simulink model "gtm_aeromodel"  (Simulink 7.2)
settings: Solver=ode45  StartTime=0.0  StopTime=10.0  RelTol=1e-3
undefined symbols (not defined in the file or in its folder): A_BLCG, A_BW, A_CW, A_FSCG, A_FSREF_in, A_SW, A_WLCG, A_WLREF, ALPHA0, bclowb, bclowbx_FMACH, bcmowb, bcmowbx_FHP, bcmowby_FMACH, cda, cdax_FLPDEF, cddr, cddrx_FMACH, cdo, cdox_FLPDEF, cdt1, cdt1x_mach, cdt2, cdt2x_mach, cdto, cdtox_mach, cdwb, cdwbx_FALPHA, cdwby_FMACH, clat, clatfr, clatfrx_FHP, clatfry_FMACH, clatx_mach, clawbfr, clawbfrx_FHP, clawbfry_FMACH, cldefr, cldefrx_FHP, cldefry_FMACH, cldtab, cldtabx_FMACH, clqwb, clqwbfr, clqwbfrx_FHP, clqwbfry_FMACH, clqwbx_mach, cltdd, cltddx_FHP, cltddy_FMACH, clwb, clwbtdd, clwbtddx_FHP, clwbtddy_FMACH, clwbx_FALPHA, clwby_FMACH, clwbzdd, clwbzddx_FHP, clwbzddy_FMACH, clzdd ... (+196)
libraries: model_lib x1
(part 6 of 10)

== system gtm_aeromodel/get aero forces and moments/AERODYNAMICS/Moment Coefficients/ROLL/CRR ==
  mach : Inport  OutDataType=sfix(16)  OutScaling=2^0
  alpha : Inport  Port=2  OutDataType=sfix(16)  OutScaling=2^0
  altitude : Inport  Port=3  OutDataType=sfix(16)  OutScaling=2^0
  flex : Inport  Port=4  OutDataType=sfix(16)  OutScaling=2^0
  rhat : Inport  Port=5  OutDataType=sfix(16)  OutScaling=2^0
  CRRFLEX : Subsystem  TreatAsAtomicUnit=on
  Fcn28 : Fcn  Expr=1/u
  Product2 : Product  Inputs=5  OutDataType=sfix(16)  OutScaling=2^0  SaturateOnIntegerOverflow=on  RndMeth=Zero  InputSameDT=on  OutDataTypeStr=Inherit: Same as first input
  Switch7 : Switch  Threshold=0.5  SaturateOnIntegerOverflow=on  InputSameDT=on
  constant : Constant  OutDataType=sfix(16)  OutScaling=2^0
  constant2 : Constant  Value=2  OutDataType=sfix(16)  OutScaling=2^0
  constant3 : Constant  Value=constants.r2d  OutDataType=sfix(16)  OutScaling=2^0
  crrtail : Product  OutDataType=sfix(16)  OutScaling=2^0  SaturateOnIntegerOverflow=on  RndMeth=Zero  InputSameDT=on  OutDataTypeStr=Inherit: Same as first input
  crrtot : Sum  Inputs=|++  OutDataType=sfix(16)  OutScaling=2^0  SaturateOnIntegerOverflow=on  InputSameDT=on  OutDataTypeStr=Inherit: Same as first input
  crrwb : Product  OutDataType=sfix(16)  OutScaling=2^0  SaturateOnIntegerOverflow=on  RndMeth=Zero  InputSameDT=on  OutDataTypeStr=Inherit: Same as first input
  crrwb_ : Subsystem  mask(2-D Table){y=crrwbx_FALPHA, z=crrwby_FMACH, tab=crrwb}
      mask prompts: y "Y vector:"; z "Z vector:"; tab "Table:"
      mask help: 2-D Table Look Up. Enter monotonic Y and Z vectors and a matrix of 2-D tables. See the help for more info.
      mask Help: The Y and Z vectors must be monotonic.  Y  indexes into the columns of the 2-D table & Z indexes into the rows of the 2-D tables.   The input values are y and z respectively (e.g., top port = y).
      mask Display: plot(-10,-10,110,110,[90,50,10],[90,40,30],[90,50,10],[50,26,20],[90,50,10],[22,13,10])
  dcyrt : Product  OutDataType=sfix(16)  OutScaling=2^0  SaturateOnIntegerOverflow=on  RndMeth=Zero  InputSameDT=on  OutDataTypeStr=Inherit: Same as first input
  rcnbvt : Subsystem  mask(2-D Table){y=cnbvtx_FMACH, z=cnbvty_FALPHA, tab=cnbvt}
      mask prompts: y "Y vector:"; z "Z vector:"; tab "Table:"
      mask help: 2-D Table Look Up. Enter monotonic Y and Z vectors and a matrix of 2-D tables. See the help for more info.
      mask Help: The Y and Z vectors must be monotonic.  Y  indexes into the columns of the 2-D table & Z indexes into the rows of the 2-D tables.   The input values are y and z respectively (e.g., top port = y).
      mask Display: plot(-10,-10,110,110,[90,50,10],[90,40,30],[90,50,10],[50,26,20],[90,50,10],[22,13,10])
  rcrbvt : Subsystem  mask(2-D Table){y=crbvtx_FMACH, z=crbvty_FALPHA, tab=crbvt}
      mask prompts: y "Y vector:"; z "Z vector:"; tab "Table:"
      mask help: 2-D Table Look Up. Enter monotonic Y and Z vectors and a matrix of 2-D tables. See the help for more info.
      mask Help: The Y and Z vectors must be monotonic.  Y  indexes into the columns of the 2-D table & Z indexes into the rows of the 2-D tables.   The input values are y and z respectively (e.g., top port = y).
      mask Display: plot(-10,-10,110,110,[90,50,10],[90,40,30],[90,50,10],[50,26,20],[90,50,10],[22,13,10])
  rcybvt : Subsystem  mask(2-D Table){y=cybvtx_FMACH, z=cybvty_FALPHA, tab=cybvt}
      mask prompts: y "Y vector:"; z "Z vector:"; tab "Table:"
      mask help: 2-D Table Look Up. Enter monotonic Y and Z vectors and a matrix of 2-D tables. See the help for more info.
      mask Help: The Y and Z vectors must be monotonic.  Y  indexes into the columns of the 2-D table & Z indexes into the rows of the 2-D tables.   The input values are y and z respectively (e.g., top port = y).
      mask Display: plot(-10,-10,110,110,[90,50,10],[90,40,30],[90,50,10],[50,26,20],[90,50,10],[22,13,10])
  dcrrhat : Outport  OutDataType=sfix(16)  OutScaling=2^0  InitialOutput=0
  wires:
  dcyrt/1 -> dcrrhat/1
  Switch7/1 -> crrwb/2, crrtail/2
  crrwb/1 -> crrtot/2
  crrwb_/1(Interp Value) -> crrwb/1
  rhat/1 -> dcyrt/2
  crrtot/1 -> dcyrt/1
  CRRFLEX/1(crrfr) -> Switch7/1
  constant/1 -> Switch7/3
  Product2/1 -> crrtail/1
  constant3/1 -> Product2/1
  rcrbvt/1(Interp Value) -> Product2/5
  Fcn28/1 -> Product2/3
  rcnbvt/1(Interp Value) -> Product2/2
  alpha/1 -> rcrbvt/2(Z), crrwb_/1(Y), rcybvt/2(Z), rcnbvt/2(Z)
  altitude/1 -> CRRFLEX/1(altitude)
  flex/1 -> CRRFLEX/Enable, Switch7/2
  mach/1 -> rcrbvt/1(Y), CRRFLEX/2(Mach), crrwb_/2(Z), rcnbvt/1(Y), rcybvt/1(Y)
  constant2/1 -> Product2/4
  rcybvt/1(Interp Value) -> Fcn28/1
  crrtail/1 -> crrtot/1

== system gtm_aeromodel/get aero forces and moments/AERODYNAMICS/Moment Coefficients/ROLL/CRRUD ==
  alpha : Inport  OutDataType=sfix(16)  OutScaling=2^0
  rud : Inport  Port=2  OutDataType=sfix(16)  OutScaling=2^0
  altitude : Inport  Port=3  OutDataType=sfix(16)  OutScaling=2^0
  flex : Inport  Port=4  OutDataType=sfix(16)  OutScaling=2^0
  mach : Inport  Port=5  OutDataType=sfix(16)  OutScaling=2^0
  CRFLEX : Subsystem  TreatAsAtomicUnit=on
  Product : Product  Inputs=3  OutDataType=sfix(16)  OutScaling=2^0  SaturateOnIntegerOverflow=on  RndMeth=Zero  InputSameDT=on  OutDataTypeStr=Inherit: Same as first input
  Switch7 : Switch  Threshold=0.5  SaturateOnIntegerOverflow=on  InputSameDT=on
  constant : Constant  OutDataType=sfix(16)  OutScaling=2^0
  crdr : Subsystem  mask(1-D Table){z=crdrx_FALPHA, tab=crdr}
      mask prompts: z "Z vector:"; tab "Table:"
      mask help: 1-D Table Look Up. Enter monotonic Z vector amd table. See the help for more info.
      mask Help: The Z vector must be monotonic.  Z indexes into the columns of the 1-D tables.   Table does not extrapolate beyound the break vectors
      mask Display: plot(@2)
  crrud : Outport  OutDataType=sfix(16)  OutScaling=2^0  InitialOutput=0
  wires:
  mach/1 -> CRFLEX/2(Mach)
  alpha/1 -> crdr/1(Z)
  crdr/1(Interp Value) -> Product/1
  rud/1 -> Product/2
  altitude/1 -> CRFLEX/1(altitude)
  Product/1 -> crrud/1
  Switch7/1 -> Product/3
  flex/1 -> CRFLEX/Enable, Switch7/2
  CRFLEX/1(crdrfr) -> Switch7/1
  constant/1 -> Switch7/3

== system gtm_aeromodel/get aero forces and moments/AERODYNAMICS/Moment Coefficients/ROLL/CRSPOIL ==
  dsb : Inport  OutDataType=sfix(16)  OutScaling=2^0
  dsl : Inport  Port=2  OutDataType=sfix(16)  OutScaling=2^0
  alpha : Inport  Port=3  OutDataType=sfix(16)  OutScaling=2^0
  mach : Inport  Port=4  OutDataType=sfix(16)  OutScaling=2^0
  flap : Inport  Port=5  OutDataType=sfix(16)  OutScaling=2^0
  altitude : Inport  Port=6  OutDataType=sfix(16)  OutScaling=2^0
  flex : Inport  Port=7  OutDataType=sfix(16)  OutScaling=2^0
  dsr : Inport  Port=8  OutDataType=sfix(16)  OutScaling=2^0
  MACH : Constant  Value=.178  OutDataType=sfix(16)  OutScaling=2^0
  Sum1 : Sum  Inputs=-+  OutDataType=sfix(16)  OutScaling=2^0  SaturateOnIntegerOverflow=on  InputSameDT=on  OutDataTypeStr=Inherit: Same as first input
  Sum10 : Sum  OutDataType=sfix(16)  OutScaling=2^0  SaturateOnIntegerOverflow=on  InputSameDT=on  OutDataTypeStr=Inherit: Same as first input
  Sum2 : Sum  Inputs=-+  OutDataType=sfix(16)  OutScaling=2^0  SaturateOnIntegerOverflow=on  InputSameDT=on  OutDataTypeStr=Inherit: Same as first input
  Sum{5..8} (4 alike) : Sum  Inputs=+-  OutDataType=sfix(16)  OutScaling=2^0  SaturateOnIntegerOverflow=on  InputSameDT=on  OutDataTypeStr=Inherit: Same as first input
  Sum9 : Sum  Inputs=-+  OutDataType=sfix(16)  OutScaling=2^0  SaturateOnIntegerOverflow=on  InputSameDT=on  OutDataTypeStr=Inherit: Same as first input
  Switch8 : Switch  Threshold=0.5  SaturateOnIntegerOverflow=on  InputSameDT=on
  Switch9 : Switch  Threshold=0.5  SaturateOnIntegerOverflow=on  InputSameDT=on
  cr_sp_fl : Subsystem  TreatAsAtomicUnit=on
  cr_sp_flex : Subsystem  TreatAsAtomicUnit=on
  dcrds : Product  OutDataType=sfix(16)  OutScaling=2^0  SaturateOnIntegerOverflow=on  RndMeth=Zero  InputSameDT=on  OutDataTypeStr=Inherit: Same as first input
  dcrwbdsbp : Subsystem  mask(1-2-3 Table){@1=dcrwbdslx_DSL, @2=dcrwbdsly_FALPHA, @3=dcrwbdslz_FMACH, @4=dcrwbdsl}
      mask prompts: @1 "X vector:"; @2 "Y vector:"; @3 "Z vector:"; @4 "Table:"
      mask help: 3-D Table Look Up. Enter monotonic X, Y and Z vectors and a matrix of 2-D tables. See the help for more info.
      mask init:
      | x=@1;y=@2;z=@3;tab=@4;
      mask Help: The X, Y and Z vectors must be monotonic.   The 3-D table is a horizontal concatenation of  2-D tables.  X  indexes into the columns of the 2-D tables & Y indexes into the rows of the 2-D tables.  Z indexes into the table levels (starting with the 1st 2-D table).   The input values are x, y and z respectively (e.g., top port = x).
      mask Display: plot([0 2 2 0 0],[0 0 2 2 0],[0 2 2.9 0.95 0],[2 2 2.7 2.7 2],[2 2.9 2.9 2 2],[0 0.85 2.7 2 0])
  dcrwbdsl : Subsystem  mask(1-2-3 Table){@1=dcrwbdslx_DSL, @2=dcrwbdsly_FALPHA, @3=dcrwbdslz_FMACH, @4=dcrwbdsl}
      mask prompts: @1 "X vector:"; @2 "Y vector:"; @3 "Z vector:"; @4 "Table:"
      mask help: 3-D Table Look Up. Enter monotonic X, Y and Z vectors and a matrix of 2-D tables. See the help for more info.
      mask init:
      | x=@1;y=@2;z=@3;tab=@4;
      mask Help: The X, Y and Z vectors must be monotonic.   The 3-D table is a horizontal concatenation of  2-D tables.  X  indexes into the columns of the 2-D tables & Y indexes into the rows of the 2-D tables.  Z indexes into the table levels (starting with the 1st 2-D table).   The input values are x, y and z respectively (e.g., top port = x).
      mask Display: plot([0 2 2 0 0],[0 0 2 2 0],[0 2 2.9 0.95 0],[2 2 2.7 2.7 2],[2 2.9 2.9 2 2],[0 0.85 2.7 2 0])
  dcrwbdsl1 : Subsystem  mask(1-2-3 Table){@1=dcrwbdslx_DSL, @2=dcrwbdsly_FALPHA, @3=dcrwbdslz_FMACH, @4=dcrwbdsl}
      mask prompts: @1 "X vector:"; @2 "Y vector:"; @3 "Z vector:"; @4 "Table:"
      mask help: 3-D Table Look Up. Enter monotonic X, Y and Z vectors and a matrix of 2-D tables. See the help for more info.
      mask init:
      | x=@1;y=@2;z=@3;tab=@4;
      mask Help: The X, Y and Z vectors must be monotonic.   The 3-D table is a horizontal concatenation of  2-D tables.  X  indexes into the columns of the 2-D tables & Y indexes into the rows of the 2-D tables.  Z indexes into the table levels (starting with the 1st 2-D table).   The input values are x, y and z respectively (e.g., top port = x).
      mask Display: plot([0 2 2 0 0],[0 0 2 2 0],[0 2 2.9 0.95 0],[2 2 2.7 2.7 2],[2 2.9 2.9 2 2],[0 0.85 2.7 2 0])
  dcrwbdsl2 : Subsystem  mask(1-2-3 Table){@1=dcrwbdslx_DSL, @2=dcrwbdsly_FALPHA, @3=dcrwbdslz_FMACH, @4=dcrwbdsl}
      mask prompts: @1 "X vector:"; @2 "Y vector:"; @3 "Z vector:"; @4 "Table:"
      mask help: 3-D Table Look Up. Enter monotonic X, Y and Z vectors and a matrix of 2-D tables. See the help for more info.
      mask init:
      | x=@1;y=@2;z=@3;tab=@4;
      mask Help: The X, Y and Z vectors must be monotonic.   The 3-D table is a horizontal concatenation of  2-D tables.  X  indexes into the columns of the 2-D tables & Y indexes into the rows of the 2-D tables.  Z indexes into the table levels (starting with the 1st 2-D table).   The input values are x, y and z respectively (e.g., top port = x).
      mask Display: plot([0 2 2 0 0],[0 0 2 2 0],[0 2 2.9 0.95 0],[2 2 2.7 2.7 2],[2 2.9 2.9 2 2],[0 0.85 2.7 2 0])
  dcrwbdsl3 : Subsystem  mask(1-2-3 Table){@1=dcrwbdslx_DSL, @2=dcrwbdsly_FALPHA, @3=dcrwbdslz_FMACH, @4=dcrwbdsl}
      mask prompts: @1 "X vector:"; @2 "Y vector:"; @3 "Z vector:"; @4 "Table:"
      mask help: 3-D Table Look Up. Enter monotonic X, Y and Z vectors and a matrix of 2-D tables. See the help for more info.
      mask init:
      | x=@1;y=@2;z=@3;tab=@4;
      mask Help: The X, Y and Z vectors must be monotonic.   The 3-D table is a horizontal concatenation of  2-D tables.  X  indexes into the columns of the 2-D tables & Y indexes into the rows of the 2-D tables.  Z indexes into the table levels (starting with the 1st 2-D table).   The input values are x, y and z respectively (e.g., top port = x).
      mask Display: plot([0 2 2 0 0],[0 0 2 2 0],[0 2 2.9 0.95 0],[2 2 2.7 2.7 2],[2 2.9 2.9 2 2],[0 0.85 2.7 2 0])
  dcrwbdsl4 : Subsystem  mask(1-2-3 Table){@1=dcrwbdslx_DSL, @2=dcrwbdsly_FALPHA, @3=dcrwbdslz_FMACH, @4=dcrwbdsl}
      mask prompts: @1 "X vector:"; @2 "Y vector:"; @3 "Z vector:"; @4 "Table:"
      mask help: 3-D Table Look Up. Enter monotonic X, Y and Z vectors and a matrix of 2-D tables. See the help for more info.
      mask init:
      | x=@1;y=@2;z=@3;tab=@4;
      mask Help: The X, Y and Z vectors must be monotonic.   The 3-D table is a horizontal concatenation of  2-D tables.  X  indexes into the columns of the 2-D tables & Y indexes into the rows of the 2-D tables.  Z indexes into the table levels (starting with the 1st 2-D table).   The input values are x, y and z respectively (e.g., top port = x).
      mask Display: plot([0 2 2 0 0],[0 0 2 2 0],[0 2 2.9 0.95 0],[2 2 2.7 2.7 2],[2 2.9 2.9 2 2],[0 0.85 2.7 2 0])
  one : Constant  Value=1.0  OutDataType=sfix(16)  OutScaling=2^0
  zero : Constant  Value=0.0  OutDataType=sfix(16)  OutScaling=2^0
  cr_spoil : Outport  OutDataType=sfix(16)  OutScaling=2^0  InitialOutput=0
  wires:
  dcrwbdsl/1(Interp Value) -> Sum1/2
  Sum10/1 -> cr_spoil/1
  alpha/1 -> dcrwbdsbp/2(Y), dcrwbdsl/2(Y), dcrwbdsl1/2(Y), dcrwbdsl3/2(Y), cr_sp_fl/2(alpha), dcrwbdsl4/2(Y), dcrwbdsl2/2(Y)
  dsl/1 -> dcrwbdsl/1(X), cr_sp_fl/3(dsl), dcrwbdsl3/1(X)
  dsb/1 -> dcrwbdsbp/1(X), cr_sp_fl/4(dsb), dcrwbdsl2/1(X)
  mach/1 -> dcrwbdsbp/3(Z), cr_sp_flex/2(mach), dcrwbdsl1/3(Z), dcrwbdsl/3(Z)
  altitude/1 -> cr_sp_flex/1(altitude)
  flap/1 -> cr_sp_fl/1(flap), cr_sp_fl/Enable, Switch8/2
  dcrwbdsl1/1(Interp Value) -> Sum5/1
  dcrwbdsbp/1(Interp Value) -> Sum1/1, Sum5/2
  Sum5/1 -> Sum6/2
  Sum6/1 -> dcrds/1
  dsr/1 -> dcrwbdsl1/1(X), dcrwbdsl4/1(X), cr_sp_fl/5(dsr)
  dcrwbdsl3/1(Interp Value) -> Sum2/2
  dcrwbdsl4/1(Interp Value) -> Sum7/1
  dcrwbdsl2/1(Interp Value) -> Sum2/1, Sum7/2
  Sum2/1 -> Sum8/1
  Sum7/1 -> Sum8/2
  MACH/1 -> dcrwbdsl2/3(Z), dcrwbdsl3/3(Z), dcrwbdsl4/3(Z)
  zero/1 -> Switch8/3
  cr_sp_fl/1(cr_sp_fl) -> Sum9/2
  Sum8/1 -> Sum9/1
  Sum9/1 -> Switch8/1
  Sum1/1 -> Sum6/1
  dcrds/1 -> Sum10/1
  Switch8/1 -> Sum10/2
  cr_sp_flex/1(cr_sp_flex) -> Switch9/1
  one/1 -> Switch9/3
  flex/1 -> cr_sp_flex/Enable, Switch9/2
  Switch9/1 -> dcrds/2

== system gtm_aeromodel/get aero forces and moments/AERODYNAMICS/Moment Coefficients/ROLL/TAIL ==
  mach : Inport  OutDataType=sfix(16)  OutScaling=2^0
  alpha : Inport  Port=2  OutDataType=sfix(16)  OutScaling=2^0
  Sum : Sum  OutDataType=sfix(16)  OutScaling=2^0  SaturateOnIntegerOverflow=on  InputSameDT=on  OutDataTypeStr=Inherit: Same as first input
  crbht : Subsystem  mask(2-D Table){y=crbhtx_FMACH, z=crbhty_FALPHA, tab=crbht}
      mask prompts: y "Y vector:"; z "Z vector:"; tab "Table:"
      mask help: 2-D Table Look Up. Enter monotonic Y and Z vectors and a matrix of 2-D tables. See the help for more info.
      mask Help: The Y and Z vectors must be monotonic.  Y  indexes into the columns of the 2-D table & Z indexes into the rows of the 2-D tables.   The input values are y and z respectively (e.g., top port = y).
      mask Display: plot(-10,-10,110,110,[90,50,10],[90,40,30],[90,50,10],[50,26,20],[90,50,10],[22,13,10])
  crbvt : Subsystem  mask(2-D Table){y=crbvtx_FMACH, z=crbvty_FALPHA, tab=crbvt}
      mask prompts: y "Y vector:"; z "Z vector:"; tab "Table:"
      mask help: 2-D Table Look Up. Enter monotonic Y and Z vectors and a matrix of 2-D tables. See the help for more info.
      mask Help: The Y and Z vectors must be monotonic.  Y  indexes into the columns of the 2-D table & Z indexes into the rows of the 2-D tables.   The input values are y and z respectively (e.g., top port = y).
      mask Display: plot(-10,-10,110,110,[90,50,10],[90,40,30],[90,50,10],[50,26,20],[90,50,10],[22,13,10])
  crt : Outport  OutDataType=sfix(16)  OutScaling=2^0  InitialOutput=0
  wires:
  crbvt/1(Interp Value) -> Sum/2
  Sum/1 -> crt/1
  crbht/1(Interp Value) -> Sum/1
  mach/1 -> crbht/1(Y), crbvt/1(Y)
  alpha/1 -> crbht/2(Z), crbvt/2(Z)

== system gtm_aeromodel/get aero forces and moments/AERODYNAMICS/Moment Coefficients/YAW/CNBWB ==
  alpha : Inport  OutDataType=sfix(16)  OutScaling=2^0
  mach : Inport  Port=2  OutDataType=sfix(16)  OutScaling=2^0
  flap : Inport  Port=3  OutDataType=sfix(16)  OutScaling=2^0
  flex : Inport  Port=4  OutDataType=sfix(16)  OutScaling=2^0
  altitude : Inport  Port=5  OutDataType=sfix(16)  OutScaling=2^0
  CNWBFLEX : Subsystem  TreatAsAtomicUnit=on
  Sum : Sum  OutDataType=sfix(16)  OutScaling=2^0  SaturateOnIntegerOverflow=on  InputSameDT=on  OutDataTypeStr=Inherit: Same as first input
  Switch5 : Switch  Threshold=0.1  SaturateOnIntegerOverflow=on  InputSameDT=on
  cn_flap_ : Subsystem  TreatAsAtomicUnit=on
  cnbwb_ : Subsystem  mask(2-D Table){y=cnbwbx_FMACH, z=cnbwby_FALPHA, tab=cnbwb}
      mask prompts: y "Y vector:"; z "Z vector:"; tab "Table:"
      mask help: 2-D Table Look Up. Enter monotonic Y and Z vectors and a matrix of 2-D tables. See the help for more info.
      mask Help: The Y and Z vectors must be monotonic.  Y  indexes into the columns of the 2-D table & Z indexes into the rows of the 2-D tables.   The input values are y and z respectively (e.g., top port = y).
      mask Display: plot(-10,-10,110,110,[90,50,10],[90,40,30],[90,50,10],[50,26,20],[90,50,10],[22,13,10])
  constant : Constant  Value=0.0  OutDataType=sfix(16)  OutScaling=2^0
  cnbwb : Outport  OutDataType=sfix(16)  OutScaling=2^0  InitialOutput=0
  cnbfr : Outport  Port=2  OutDataType=sfix(16)  OutScaling=2^0  InitialOutput=0
  wires:
  alpha/1 -> cn_flap_/2(alpha), cnbwb_/2(Z)
  Sum/1 -> cnbwb/1
  cnbwb_/1(Interp Value) -> Sum/2
  flap/1 -> cn_flap_/1(flap), cn_flap_/Enable, Switch5/2
  cn_flap_/1(cn_flap) -> Switch5/1
  altitude/1 -> CNWBFLEX/1(altitude)
  mach/1 -> cnbwb_/1(Y), CNWBFLEX/2(Mach)
  constant/1 -> Switch5/3
  Switch5/1 -> Sum/1
  flex/1 -> CNWBFLEX/Enable
  CNWBFLEX/1(cnbfr) -> cnbfr/1

== system gtm_aeromodel/get aero forces and moments/AERODYNAMICS/Moment Coefficients/YAW/CNGEAR ==
  flap : Inport  OutDataType=sfix(16)  OutScaling=2^0
  gear : Inport  Port=2  OutDataType=sfix(16)  OutScaling=2^0
  beta : Inport  Port=3  OutDataType=sfix(16)  OutScaling=2^0
  Product1 : Product  OutDataType=sfix(16)  OutScaling=2^0  SaturateOnIntegerOverflow=on  RndMeth=Zero  InputSameDT=on  OutDataTypeStr=Inherit: Same as first input
  Switch6 : Switch  Threshold=0.5  SaturateOnIntegerOverflow=on  InputSameDT=on
  constant1 : Constant  Value=0.0  OutDataType=sfix(16)  OutScaling=2^0
  dcnb : Subsystem  mask(1-D Table){z=dcnbx_FLPDEF, tab=dcnb}
      mask prompts: z "Z vector:"; tab "Table:"
      mask help: 1-D Table Look Up. Enter monotonic Z vector amd table. See the help for more info.
      mask Help: The Z vector must be monotonic.  Z indexes into the columns of the 1-D tables.   Table does not extrapolate beyound the break vectors
      mask Display: plot(@2)
  cng : Outport  OutDataType=sfix(16)  OutScaling=2^0  InitialOutput=0
  wires:
  Product1/1 -> Switch6/1
  beta/1 -> Product1/1
  Switch6/1 -> cng/1
  constant1/1 -> Switch6/3
  gear/1 -> Switch6/2
  flap/1 -> dcnb/1(Z)
  dcnb/1(Interp Value) -> Product1/2

== system gtm_aeromodel/get aero forces and moments/AERODYNAMICS/Moment Coefficients/YAW/CNP ==
  mach : Inport  OutDataType=sfix(16)  OutScaling=2^0
  alpha : Inport  Port=2  OutDataType=sfix(16)  OutScaling=2^0
  altitude : Inport  Port=3  OutDataType=sfix(16)  OutScaling=2^0
  flex : Inport  Port=4  OutDataType=sfix(16)  OutScaling=2^0
  phat : Inport  Port=5  OutDataType=sfix(16)  OutScaling=2^0
  CNPFLEX : Subsystem  TreatAsAtomicUnit=on
  Fcn28 : Fcn  Expr=1/u
  Product2 : Product  Inputs=5  OutDataType=sfix(16)  OutScaling=2^0  SaturateOnIntegerOverflow=on  RndMeth=Zero  InputSameDT=on  OutDataTypeStr=Inherit: Same as first input
  Switch7 : Switch  Threshold=0.5  SaturateOnIntegerOverflow=on  InputSameDT=on
  cnptail : Product  OutDataType=sfix(16)  OutScaling=2^0  SaturateOnIntegerOverflow=on  RndMeth=Zero  InputSameDT=on  OutDataTypeStr=Inherit: Same as first input
  cnptot : Sum  Inputs=|++  OutDataType=sfix(16)  OutScaling=2^0  SaturateOnIntegerOverflow=on  InputSameDT=on  OutDataTypeStr=Inherit: Same as first input
  cnpwb : Product  OutDataType=sfix(16)  OutScaling=2^0  SaturateOnIntegerOverflow=on  RndMeth=Zero  InputSameDT=on  OutDataTypeStr=Inherit: Same as first input
  constant : Constant  OutDataType=sfix(16)  OutScaling=2^0
  constant2 : Constant  Value=2  OutDataType=sfix(16)  OutScaling=2^0
  constant3 : Constant  Value=constants.r2d  OutDataType=sfix(16)  OutScaling=2^0
  dcyrt : Product  OutDataType=sfix(16)  OutScaling=2^0  SaturateOnIntegerOverflow=on  RndMeth=Zero  InputSameDT=on  OutDataTypeStr=Inherit: Same as first input
  rcnbvt : Subsystem  mask(2-D Table){y=cnbvtx_FMACH, z=cnbvty_FALPHA, tab=cnbvt}
      mask prompts: y "Y vector:"; z "Z vector:"; tab "Table:"
      mask help: 2-D Table Look Up. Enter monotonic Y and Z vectors and a matrix of 2-D tables. See the help for more info.
      mask Help: The Y and Z vectors must be monotonic.  Y  indexes into the columns of the 2-D table & Z indexes into the rows of the 2-D tables.   The input values are y and z respectively (e.g., top port = y).
      mask Display: plot(-10,-10,110,110,[90,50,10],[90,40,30],[90,50,10],[50,26,20],[90,50,10],[22,13,10])
  rcnpwb : Subsystem  mask(2-D Table){y=cnpwbx_FMACH, z=cnpwby_FALPHA, tab=cnpwb}
      mask prompts: y "Y vector:"; z "Z vector:"; tab "Table:"
      mask help: 2-D Table Look Up. Enter monotonic Y and Z vectors and a matrix of 2-D tables. See the help for more info.
      mask Help: The Y and Z vectors must be monotonic.  Y  indexes into the columns of the 2-D table & Z indexes into the rows of the 2-D tables.   The input values are y and z respectively (e.g., top port = y).
      mask Display: plot(-10,-10,110,110,[90,50,10],[90,40,30],[90,50,10],[50,26,20],[90,50,10],[22,13,10])
  rcrbvt : Subsystem  mask(2-D Table){y=crbvtx_FMACH, z=crbvty_FALPHA, tab=crbvt}
      mask prompts: y "Y vector:"; z "Z vector:"; tab "Table:"
      mask help: 2-D Table Look Up. Enter monotonic Y and Z vectors and a matrix of 2-D tables. See the help for more info.
      mask Help: The Y and Z vectors must be monotonic.  Y  indexes into the columns of the 2-D table & Z indexes into the rows of the 2-D tables.   The input values are y and z respectively (e.g., top port = y).
      mask Display: plot(-10,-10,110,110,[90,50,10],[90,40,30],[90,50,10],[50,26,20],[90,50,10],[22,13,10])
  rcybvt : Subsystem  mask(2-D Table){y=cybvtx_FMACH, z=cybvty_FALPHA, tab=cybvt}
      mask prompts: y "Y vector:"; z "Z vector:"; tab "Table:"
      mask help: 2-D Table Look Up. Enter monotonic Y and Z vectors and a matrix of 2-D tables. See the help for more info.
      mask Help: The Y and Z vectors must be monotonic.  Y  indexes into the columns of the 2-D table & Z indexes into the rows of the 2-D tables.   The input values are y and z respectively (e.g., top port = y).
      mask Display: plot(-10,-10,110,110,[90,50,10],[90,40,30],[90,50,10],[50,26,20],[90,50,10],[22,13,10])
  dcnphat : Outport  Orientation=left  OutDataType=sfix(16)  OutScaling=2^0  InitialOutput=0
  wires:
  constant3/1 -> Product2/1
  rcnbvt/1(Interp Value) -> Product2/5
  rcybvt/1(Interp Value) -> Fcn28/1
  rcrbvt/1(Interp Value) -> Product2/2
  Switch7/1 -> cnpwb/2, cnptail/2
  cnpwb/1 -> cnptot/2
  rcnpwb/1(Interp Value) -> cnpwb/1
  constant/1 -> Switch7/3
  CNPFLEX/1(cnpfr) -> Switch7/1
  Product2/1 -> cnptail/1
  cnptot/1 -> dcyrt/1
  phat/1 -> dcyrt/2
  cnptail/1 -> cnptot/1
  constant2/1 -> Product2/4
  mach/1 -> rcnbvt/1(Y), rcnpwb/1(Y), CNPFLEX/2(Mach), rcybvt/1(Y), rcrbvt/1(Y)
  flex/1 -> Switch7/2, CNPFLEX/Enable
  altitude/1 -> CNPFLEX/1(altitude)
  alpha/1 -> rcnbvt/2(Z), rcybvt/2(Z), rcrbvt/2(Z), rcnpwb/2(Z)
  Fcn28/1 -> Product2/3
  dcyrt/1 -> dcnphat/1

== system gtm_aeromodel/get aero forces and moments/AERODYNAMICS/Moment Coefficients/YAW/CNR ==
  mach : Inport  OutDataType=sfix(16)  OutScaling=2^0
  alpha : Inport  Port=2  OutDataType=sfix(16)  OutScaling=2^0
  altitude : Inport  Port=3  OutDataType=sfix(16)  OutScaling=2^0
  flex : Inport  Port=4  OutDataType=sfix(16)  OutScaling=2^0
  rhat : Inport  Port=5  OutDataType=sfix(16)  OutScaling=2^0
  CNRFLEX : Subsystem  TreatAsAtomicUnit=on
  Fcn28 : Fcn  Expr=1/u
  Product2 : Product  Inputs=4  OutDataType=sfix(16)  OutScaling=2^0  SaturateOnIntegerOverflow=on  RndMeth=Zero  InputSameDT=on  OutDataTypeStr=Inherit: Same as first input
  Product3 : Product  OutDataType=sfix(16)  OutScaling=2^0  SaturateOnIntegerOverflow=on  RndMeth=Zero  InputSameDT=on  OutDataTypeStr=Inherit: Same as first input
  Switch7 : Switch  Threshold=0.5  SaturateOnIntegerOverflow=on  InputSameDT=on
  cnrtail : Product  OutDataType=sfix(16)  OutScaling=2^0  SaturateOnIntegerOverflow=on  RndMeth=Zero  InputSameDT=on  OutDataTypeStr=Inherit: Same as first input
  cnrtot : Sum  Inputs=|++  OutDataType=sfix(16)  OutScaling=2^0  SaturateOnIntegerOverflow=on  InputSameDT=on  OutDataTypeStr=Inherit: Same as first input
  cnrwb : Product  OutDataType=sfix(16)  OutScaling=2^0  SaturateOnIntegerOverflow=on  RndMeth=Zero  InputSameDT=on  OutDataTypeStr=Inherit: Same as first input
  constant : Constant  OutDataType=sfix(16)  OutScaling=2^0
  constant2 : Constant  Value=2  OutDataType=sfix(16)  OutScaling=2^0
  constant3 : Constant  Value=constants.r2d  OutDataType=sfix(16)  OutScaling=2^0
  dcyrt : Product  OutDataType=sfix(16)  OutScaling=2^0  SaturateOnIntegerOverflow=on  RndMeth=Zero  InputSameDT=on  OutDataTypeStr=Inherit: Same as first input
  rcnbvt : Subsystem  mask(2-D Table){y=cnbvtx_FMACH, z=cnbvty_FALPHA, tab=cnbvt}
      mask prompts: y "Y vector:"; z "Z vector:"; tab "Table:"
      mask help: 2-D Table Look Up. Enter monotonic Y and Z vectors and a matrix of 2-D tables. See the help for more info.
      mask Help: The Y and Z vectors must be monotonic.  Y  indexes into the columns of the 2-D table & Z indexes into the rows of the 2-D tables.   The input values are y and z respectively (e.g., top port = y).
      mask Display: plot(-10,-10,110,110,[90,50,10],[90,40,30],[90,50,10],[50,26,20],[90,50,10],[22,13,10])
  rcnrwb : Subsystem  mask(2-D Table){y=cnrwbx_FALPHA, z=cnrwby_FMACH, tab=cnrwb}
      mask prompts: y "Y vector:"; z "Z vector:"; tab "Table:"
      mask help: 2-D Table Look Up. Enter monotonic Y and Z vectors and a matrix of 2-D tables. See the help for more info.
      mask Help: The Y and Z vectors must be monotonic.  Y  indexes into the columns of the 2-D table & Z indexes into the rows of the 2-D tables.   The input values are y and z respectively (e.g., top port = y).
      mask Display: plot(-10,-10,110,110,[90,50,10],[90,40,30],[90,50,10],[50,26,20],[90,50,10],[22,13,10])
  rcybvt : Subsystem  mask(2-D Table){y=cybvtx_FMACH, z=cybvty_FALPHA, tab=cybvt}
      mask prompts: y "Y vector:"; z "Z vector:"; tab "Table:"
      mask help: 2-D Table Look Up. Enter monotonic Y and Z vectors and a matrix of 2-D tables. See the help for more info.
      mask Help: The Y and Z vectors must be monotonic.  Y  indexes into the columns of the 2-D table & Z indexes into the rows of the 2-D tables.   The input values are y and z respectively (e.g., top port = y).
      mask Display: plot(-10,-10,110,110,[90,50,10],[90,40,30],[90,50,10],[50,26,20],[90,50,10],[22,13,10])
  dcnrhat : Outport  OutDataType=sfix(16)  OutScaling=2^0  InitialOutput=0
  wires:
  constant3/1 -> Product2/1
  Switch7/1 -> cnrwb/2, cnrtail/2
  constant/1 -> Switch7/3
  CNRFLEX/1(cnrfr) -> Switch7/1
  Product3/1 -> Product2/2
  rcnbvt/1(Interp Value) -> Product3/2, Product3/1
  cnrwb/1 -> cnrtot/2
  rcnrwb/1(Interp Value) -> cnrwb/1
  Product2/1 -> cnrtail/1
  dcyrt/1 -> dcnrhat/1
  cnrtot/1 -> dcyrt/1
  rhat/1 -> dcyrt/2
  cnrtail/1 -> cnrtot/1
  rcybvt/1(Interp Value) -> Fcn28/1
  constant2/1 -> Product2/4
  mach/1 -> rcnrwb/2(Z), CNRFLEX/2(Mach), rcybvt/1(Y), rcnbvt/1(Y)
  flex/1 -> Switch7/2, CNRFLEX/Enable
  altitude/1 -> CNRFLEX/1(altitude)
  alpha/1 -> rcnbvt/2(Z), rcybvt/2(Z), rcnrwb/1(Y)
  Fcn28/1 -> Product2/3

== system gtm_aeromodel/get aero forces and moments/AERODYNAMICS/Moment Coefficients/YAW/CNRUD ==
  rud : Inport  OutDataType=sfix(16)  OutScaling=2^0
  altitude : Inport  Port=2  OutDataType=sfix(16)  OutScaling=2^0
  flex : Inport  Port=3  OutDataType=sfix(16)  OutScaling=2^0
  mach : Inport  Port=4  OutDataType=sfix(16)  OutScaling=2^0
  CNFLEX : Subsystem  TreatAsAtomicUnit=on
  Product : Product  Inputs=3  OutDataType=sfix(16)  OutScaling=2^0  SaturateOnIntegerOverflow=on  RndMeth=Zero  InputSameDT=on  OutDataTypeStr=Inherit: Same as first input
  Switch7 : Switch  Threshold=0.5  SaturateOnIntegerOverflow=on  InputSameDT=on
  cndr : Subsystem  mask(1-D Table){z=cndrx_FMACH, tab=cndr}
      mask prompts: z "Z vector:"; tab "Table:"
      mask help: 1-D Table Look Up. Enter monotonic Z vector amd table. See the help for more info.
      mask Help: The Z vector must be monotonic.  Z indexes into the columns of the 1-D tables.   Table does not extrapolate beyound the break vectors
      mask Display: plot(@2)
  constant : Constant  OutDataType=sfix(16)  OutScaling=2^0
  cnrud : Outport  OutDataType=sfix(16)  OutScaling=2^0  InitialOutput=0
  wires:
  mach/1 -> cndr/1(Z), CNFLEX/2(Mach)
  constant/1 -> Switch7/3
  CNFLEX/1(cndrfr) -> Switch7/1
  flex/1 -> Switch7/2, CNFLEX/Enable
  Switch7/1 -> Product/3
  Product/1 -> cnrud/1
  altitude/1 -> CNFLEX/1(altitude)
  rud/1 -> Product/2
  cndr/1(Interp Value) -> Product/1

== system gtm_aeromodel/get aero forces and moments/AERODYNAMICS/Moment Coefficients/YAW/CNSPOIL ==
  dsb : Inport  OutDataType=sfix(16)  OutScaling=2^0
  dsl : Inport  Port=2  OutDataType=sfix(16)  OutScaling=2^0
  alpha : Inport  Port=3  OutDataType=sfix(16)  OutScaling=2^0
  mach : Inport  Port=4  OutDataType=sfix(16)  OutScaling=2^0
  flap : Inport  Port=5  OutDataType=sfix(16)  OutScaling=2^0
  dsr : Inport  Port=6  OutDataType=sfix(16)  OutScaling=2^0
  MACH : Constant  Value=.178  OutDataType=sfix(16)  OutScaling=2^0
  Sum1 : Sum  Inputs=-+  OutDataType=sfix(16)  OutScaling=2^0  SaturateOnIntegerOverflow=on  InputSameDT=on  OutDataTypeStr=Inherit: Same as first input
  Sum10 : Sum  OutDataType=sfix(16)  OutScaling=2^0  SaturateOnIntegerOverflow=on  InputSameDT=on  OutDataTypeStr=Inherit: Same as first input
  Sum2 : Sum  Inputs=-+  OutDataType=sfix(16)  OutScaling=2^0  SaturateOnIntegerOverflow=on  InputSameDT=on  OutDataTypeStr=Inherit: Same as first input
  Sum{5..8} (4 alike) : Sum  Inputs=+-  OutDataType=sfix(16)  OutScaling=2^0  SaturateOnIntegerOverflow=on  InputSameDT=on  OutDataTypeStr=Inherit: Same as first input
  Sum9 : Sum  Inputs=-+  OutDataType=sfix(16)  OutScaling=2^0  SaturateOnIntegerOverflow=on  InputSameDT=on  OutDataTypeStr=Inherit: Same as first input
  Switch8 : Switch  Threshold=0.5  SaturateOnIntegerOverflow=on  InputSameDT=on
  cn_sp_fl : Subsystem  TreatAsAtomicUnit=on
  dcnwbdsl : Subsystem  mask(1-2-3 Table){@1=dcnwbdslx_DSL, @2=dcnwbdsly_FALPHA, @3=dcnwbdslz_FMACH, @4=dcnwbdsl}
      mask prompts: @1 "X vector:"; @2 "Y vector:"; @3 "Z vector:"; @4 "Table:"
      mask help: 3-D Table Look Up. Enter monotonic X, Y and Z vectors and a matrix of 2-D tables. See the help for more info.
      mask init:
      | x=@1;y=@2;z=@3;tab=@4;
      mask Help: The X, Y and Z vectors must be monotonic.   The 3-D table is a horizontal concatenation of  2-D tables.  X  indexes into the columns of the 2-D tables & Y indexes into the rows of the 2-D tables.  Z indexes into the table levels (starting with the 1st 2-D table).   The input values are x, y and z respectively (e.g., top port = x).
      mask Display: plot([0 2 2 0 0],[0 0 2 2 0],[0 2 2.9 0.95 0],[2 2 2.7 2.7 2],[2 2.9 2.9 2 2],[0 0.85 2.7 2 0])
  dcnwbdsl1 : Subsystem  mask(1-2-3 Table){@1=dcnwbdslx_DSL, @2=dcnwbdsly_FALPHA, @3=dcnwbdslz_FMACH, @4=dcnwbdsl}
      mask prompts: @1 "X vector:"; @2 "Y vector:"; @3 "Z vector:"; @4 "Table:"
      mask help: 3-D Table Look Up. Enter monotonic X, Y and Z vectors and a matrix of 2-D tables. See the help for more info.
      mask init:
      | x=@1;y=@2;z=@3;tab=@4;
      mask Help: The X, Y and Z vectors must be monotonic.   The 3-D table is a horizontal concatenation of  2-D tables.  X  indexes into the columns of the 2-D tables & Y indexes into the rows of the 2-D tables.  Z indexes into the table levels (starting with the 1st 2-D table).   The input values are x, y and z respectively (e.g., top port = x).
      mask Display: plot([0 2 2 0 0],[0 0 2 2 0],[0 2 2.9 0.95 0],[2 2 2.7 2.7 2],[2 2.9 2.9 2 2],[0 0.85 2.7 2 0])
  dcnwbdsl2 : Subsystem  mask(1-2-3 Table){@1=dcnwbdslx_DSL, @2=dcnwbdsly_FALPHA, @3=dcnwbdslz_FMACH, @4=dcnwbdsl}
      mask prompts: @1 "X vector:"; @2 "Y vector:"; @3 "Z vector:"; @4 "Table:"
      mask help: 3-D Table Look Up. Enter monotonic X, Y and Z vectors and a matrix of 2-D tables. See the help for more info.
      mask init:
      | x=@1;y=@2;z=@3;tab=@4;
      mask Help: The X, Y and Z vectors must be monotonic.   The 3-D table is a horizontal concatenation of  2-D tables.  X  indexes into the columns of the 2-D tables & Y indexes into the rows of the 2-D tables.  Z indexes into the table levels (starting with the 1st 2-D table).   The input values are x, y and z respectively (e.g., top port = x).
      mask Display: plot([0 2 2 0 0],[0 0 2 2 0],[0 2 2.9 0.95 0],[2 2 2.7 2.7 2],[2 2.9 2.9 2 2],[0 0.85 2.7 2 0])
  dcnwbdsl3 : Subsystem  mask(1-2-3 Table){@1=dcnwbdslx_DSL, @2=dcnwbdsly_FALPHA, @3=dcnwbdslz_FMACH, @4=dcnwbdsl}
      mask prompts: @1 "X vector:"; @2 "Y vector:"; @3 "Z vector:"; @4 "Table:"
      mask help: 3-D Table Look Up. Enter monotonic X, Y and Z vectors and a matrix of 2-D tables. See the help for more info.
      mask init:
      | x=@1;y=@2;z=@3;tab=@4;
      mask Help: The X, Y and Z vectors must be monotonic.   The 3-D table is a horizontal concatenation of  2-D tables.  X  indexes into the columns of the 2-D tables & Y indexes into the rows of the 2-D tables.  Z indexes into the table levels (starting with the 1st 2-D table).   The input values are x, y and z respectively (e.g., top port = x).
      mask Display: plot([0 2 2 0 0],[0 0 2 2 0],[0 2 2.9 0.95 0],[2 2 2.7 2.7 2],[2 2.9 2.9 2 2],[0 0.85 2.7 2 0])
  dcnwbdsl4 : Subsystem  mask(1-2-3 Table){@1=dcnwbdslx_DSL, @2=dcnwbdsly_FALPHA, @3=dcnwbdslz_FMACH, @4=dcnwbdsl}
      mask prompts: @1 "X vector:"; @2 "Y vector:"; @3 "Z vector:"; @4 "Table:"
      mask help: 3-D Table Look Up. Enter monotonic X, Y and Z vectors and a matrix of 2-D tables. See the help for more info.
      mask init:
      | x=@1;y=@2;z=@3;tab=@4;
      mask Help: The X, Y and Z vectors must be monotonic.   The 3-D table is a horizontal concatenation of  2-D tables.  X  indexes into the columns of the 2-D tables & Y indexes into the rows of the 2-D tables.  Z indexes into the table levels (starting with the 1st 2-D table).   The input values are x, y and z respectively (e.g., top port = x).
      mask Display: plot([0 2 2 0 0],[0 0 2 2 0],[0 2 2.9 0.95 0],[2 2 2.7 2.7 2],[2 2.9 2.9 2 2],[0 0.85 2.7 2 0])
  dcnwbdsl5 : Subsystem  mask(1-2-3 Table){@1=dcnwbdslx_DSL, @2=dcnwbdsly_FALPHA, @3=dcnwbdslz_FMACH, @4=dcnwbdsl}
      mask prompts: @1 "X vector:"; @2 "Y vector:"; @3 "Z vector:"; @4 "Table:"
      mask help: 3-D Table Look Up. Enter monotonic X, Y and Z vectors and a matrix of 2-D tables. See the help for more info.
      mask init:
      | x=@1;y=@2;z=@3;tab=@4;
      mask Help: The X, Y and Z vectors must be monotonic.   The 3-D table is a horizontal concatenation of  2-D tables.  X  indexes into the columns of the 2-D tables & Y indexes into the rows of the 2-D tables.  Z indexes into the table levels (starting with the 1st 2-D table).   The input values are x, y and z respectively (e.g., top port = x).
      mask Display: plot([0 2 2 0 0],[0 0 2 2 0],[0 2 2.9 0.95 0],[2 2 2.7 2.7 2],[2 2.9 2.9 2 2],[0 0.85 2.7 2 0])
  zero : Constant  Value=0.0  OutDataType=sfix(16)  OutScaling=2^0
  cn_spoil : Outport  Orientation=left  OutDataType=sfix(16)  OutScaling=2^0  InitialOutput=0
  wires:
  Switch8/1 -> Sum10/2
  Sum1/1 -> Sum6/1
  Sum9/1 -> Switch8/1
  Sum8/1 -> Sum9/1
  cn_sp_fl/1(cn_sp_fl) -> Sum9/2
  zero/1 -> Switch8/3
  MACH/1 -> dcnwbdsl5/3(Z), dcnwbdsl4/3(Z), dcnwbdsl3/3(Z)
  Sum7/1 -> Sum8/2
  Sum2/1 -> Sum8/1
  dcnwbdsl3/1(Interp Value) -> Sum7/2, Sum2/1
  dcnwbdsl5/1(Interp Value) -> Sum7/1
  dcnwbdsl4/1(Interp Value) -> Sum2/2
  dsr/1 -> cn_sp_fl/5(dsr), dcnwbdsl5/1(X), dcnwbdsl2/1(X)
  Sum5/1 -> Sum6/2
  dcnwbdsl/1(Interp Value) -> Sum5/2, Sum1/1
  dcnwbdsl2/1(Interp Value) -> Sum5/1
  flap/1 -> Switch8/2, cn_sp_fl/Enable, cn_sp_fl/1(flap)
  mach/1 -> dcnwbdsl1/3(Z), dcnwbdsl/3(Z), dcnwbdsl2/3(Z)
  dsb/1 -> dcnwbdsl3/1(X), cn_sp_fl/4(dsb), dcnwbdsl/1(X)
  dsl/1 -> dcnwbdsl4/1(X), cn_sp_fl/3(dsl), dcnwbdsl1/1(X)
  alpha/1 -> dcnwbdsl3/2(Y), dcnwbdsl5/2(Y), cn_sp_fl/2(alpha), dcnwbdsl4/2(Y), dcnwbdsl2/2(Y), dcnwbdsl1/2(Y), dcnwbdsl/2(Y)
  Sum10/1 -> cn_spoil/1
  dcnwbdsl1/1(Interp Value) -> Sum1/2
  Sum6/1 -> Sum10/1

== system gtm_aeromodel/get aero forces and moments/AERODYNAMICS/Moment Coefficients/YAW/CNT ==
  mach : Inport  OutDataType=sfix(16)  OutScaling=2^0
  alpha : Inport  Port=2  OutDataType=sfix(16)  OutScaling=2^0
  Sum : Sum  OutDataType=sfix(16)  OutScaling=2^0  SaturateOnIntegerOverflow=on  InputSameDT=on  OutDataTypeStr=Inherit: Same as first input
  cnbht : Subsystem  mask(2-D Table){y=cnbhtx_FMACH, z=cnbhty_FALPHA, tab=cnbht}
      mask prompts: y "Y vector:"; z "Z vector:"; tab "Table:"
      mask help: 2-D Table Look Up. Enter monotonic Y and Z vectors and a matrix of 2-D tables. See the help for more info.
      mask Help: The Y and Z vectors must be monotonic.  Y  indexes into the columns of the 2-D table & Z indexes into the rows of the 2-D tables.   The input values are y and z respectively (e.g., top port = y).
      mask Display: plot(-10,-10,110,110,[90,50,10],[90,40,30],[90,50,10],[50,26,20],[90,50,10],[22,13,10])
  cnbvt : Subsystem  mask(2-D Table){y=cnbvtx_FMACH, z=cnbvty_FALPHA, tab=cnbvt}
      mask prompts: y "Y vector:"; z "Z vector:"; tab "Table:"
      mask help: 2-D Table Look Up. Enter monotonic Y and Z vectors and a matrix of 2-D tables. See the help for more info.
      mask Help: The Y and Z vectors must be monotonic.  Y  indexes into the columns of the 2-D table & Z indexes into the rows of the 2-D tables.   The input values are y and z respectively (e.g., top port = y).
      mask Display: plot(-10,-10,110,110,[90,50,10],[90,40,30],[90,50,10],[50,26,20],[90,50,10],[22,13,10])
  cnt : Outport  OutDataType=sfix(16)  OutScaling=2^0  InitialOutput=0
  wires:
  alpha/1 -> cnbvt/2(Z), cnbht/2(Z)
  mach/1 -> cnbvt/1(Y), cnbht/1(Y)
  cnbht/1(Interp Value) -> Sum/1
  Sum/1 -> cnt/1
  cnbvt/1(Interp Value) -> Sum/2

== system gtm_aeromodel/get aero forces and moments/AERODYNAMICS/Aero Incidence Angles/DOWNWASH/deps_hob_/depshob_ ==
  X : Inport  OutDataType=sfix(16)  OutScaling=2^0
  Y : Inport  Port=2  OutDataType=sfix(16)  OutScaling=2^0
  Z : Inport  Port=3  OutDataType=sfix(16)  OutScaling=2^0
  Mux : Mux  Inputs=3
  S-Function : S-Function  FunctionName=table3v5  Parameters=x,y,z,tab  EnableBusSupport=off
  Interp Value : Outport  OutDataType=sfix(16)  OutScaling=2^0
  wires:
  Z/1 -> Mux/3
  Y/1 -> Mux/2
  X/1 -> Mux/1
  Mux/1 -> S-Function/1
  S-Function/1 -> Interp Value/1

== system gtm_aeromodel/get aero forces and moments/AERODYNAMICS/Aero Incidence Angles/DOWNWASH/depsct/gbct ==
  Z : Inport  OutDataType=sfix(16)  OutScaling=2^0
  S-Function : S-Function  FunctionName=table1v5  Parameters=z,tab  EnableBusSupport=off
  Interp Value : Outport  OutDataType=sfix(16)  OutScaling=2^0
  wires:
  Z/1 -> S-Function/1
  S-Function/1 -> Interp Value/1

== system gtm_aeromodel/get aero forces and moments/AERODYNAMICS/Aero Incidence Angles/DOWNWASH/eps_flap/dclwbdffr ==
  qdyn : Inport  OutDataType=sfix(16)  OutScaling=2^0
  flap : Inport  Port=2  OutDataType=sfix(16)  OutScaling=2^0
  Enable : EnablePort
  dclwbdffr_ : Subsystem  mask(2-D Table){y=dclwbdffrx_FQ, z=dclwbdffry_FLPDEF, tab=dclwbdffr}
      mask prompts: y "Y vector:"; z "Z vector:"; tab "Table:"
      mask help: 2-D Table Look Up. Enter monotonic Y and Z vectors and a matrix of 2-D tables. See the help for more info.
      mask Help: The Y and Z vectors must be monotonic.  Y  indexes into the columns of the 2-D table & Z indexes into the rows of the 2-D tables.   The input values are y and z respectively (e.g., top port = y).
      mask Display: plot(-10,-10,110,110,[90,50,10],[90,40,30],[90,50,10],[50,26,20],[90,50,10],[22,13,10])
  dclwbdffr : Outport  OutDataType=sfix(16)  OutScaling=2^0  InitialOutput=0
  wires:
  dclwbdffr_/1(Interp Value) -> dclwbdffr/1
  qdyn/1 -> dclwbdffr_/1(Y)
  flap/1 -> dclwbdffr_/2(Z)

== system gtm_aeromodel/get aero forces and moments/AERODYNAMICS/Aero Incidence Angles/DOWNWASH/eps_flap/epsa ==
  Z : Inport  OutDataType=sfix(16)  OutScaling=2^0
  S-Function : S-Function  FunctionName=table1v5  Parameters=z,tab  EnableBusSupport=off
  Interp Value : Outport  OutDataType=sfix(16)  OutScaling=2^0
  wires:
  S-Function/1 -> Interp Value/1
  Z/1 -> S-Function/1

== system gtm_aeromodel/get aero forces and moments/AERODYNAMICS/Aero Incidence Angles/DOWNWASH/eps_flap/epsdsbdf ==
  X : Inport  OutDataType=sfix(16)  OutScaling=2^0
  Y : Inport  Port=2  OutDataType=sfix(16)  OutScaling=2^0
  Z : Inport  Port=3  OutDataType=sfix(16)  OutScaling=2^0
  Mux : Mux  Inputs=3
  S-Function : S-Function  FunctionName=table3v5  Parameters=x,y,z,tab  EnableBusSupport=off
  Interp Value : Outport  OutDataType=sfix(16)  OutScaling=2^0
  wires:
  Z/1 -> Mux/3
  Y/1 -> Mux/2
  X/1 -> Mux/1
  Mux/1 -> S-Function/1
  S-Function/1 -> Interp Value/1

== system gtm_aeromodel/get aero forces and moments/AERODYNAMICS/Aero Incidence Angles/DOWNWASH/eps_flap/epsodsb ==
  Y : Inport  OutDataType=sfix(16)  OutScaling=2^0
  Z : Inport  Port=2  OutDataType=sfix(16)  OutScaling=2^0
  Mux : Mux  Inputs=2
  S-Function : S-Function  FunctionName=table2v5  Parameters=y,z,tab  EnableBusSupport=off
  Interp Value : Outport  OutDataType=sfix(16)  OutScaling=2^0
  wires:
  Z/1 -> Mux/2
  Y/1 -> Mux/1
  S-Function/1 -> Interp Value/1
  Mux/1 -> S-Function/1

== system gtm_aeromodel/get aero forces and moments/AERODYNAMICS/Aero Incidence Angles/DOWNWASH/eps_speedbrake_/epsodsb ==
  Y : Inport  OutDataType=sfix(16)  OutScaling=2^0
  Z : Inport  Port=2  OutDataType=sfix(16)  OutScaling=2^0
  Mux : Mux  Inputs=2
  S-Function : S-Function  FunctionName=table2v5  Parameters=y,z,tab  EnableBusSupport=off
  Interp Value : Outport  OutDataType=sfix(16)  OutScaling=2^0
  wires:
  Z/1 -> Mux/2
  Y/1 -> Mux/1
  S-Function/1 -> Interp Value/1
  Mux/1 -> S-Function/1

== system gtm_aeromodel/get aero forces and moments/AERODYNAMICS/Aero Incidence Angles/DOWNWASH/eps_speedbrake_/epsodsb_0 ==
  Y : Inport  OutDataType=sfix(16)  OutScaling=2^0
  Z : Inport  Port=2  OutDataType=sfix(16)  OutScaling=2^0
  Mux : Mux  Inputs=2
  S-Function : S-Function  FunctionName=table2v5  Parameters=y,z,tab  EnableBusSupport=off
  Interp Value : Outport  OutDataType=sfix(16)  OutScaling=2^0
  wires:
  Mux/1 -> S-Function/1
  S-Function/1 -> Interp Value/1
  Y/1 -> Mux/1
  Z/1 -> Mux/2

== system gtm_aeromodel/get aero forces and moments/AERODYNAMICS/Aero Incidence Angles/DOWNWASH/eps_spoiler_/dclsbfr_ ==
  altitude : Inport  OutDataType=sfix(16)  OutScaling=2^0
  mach : Inport  Port=2  OutDataType=sfix(16)  OutScaling=2^0
  Enable : EnablePort
  dcldsbfr : Subsystem  mask(2-D Table){y=dcldsbfrx_FHP, z=dcldsbfry_FMACH, tab=dcldsbfr}
      mask prompts: y "Y vector:"; z "Z vector:"; tab "Table:"
      mask help: 2-D Table Look Up. Enter monotonic Y and Z vectors and a matrix of 2-D tables. See the help for more info.
      mask Help: The Y and Z vectors must be monotonic.  Y  indexes into the columns of the 2-D table & Z indexes into the rows of the 2-D tables.   The input values are y and z respectively (e.g., top port = y).
      mask Display: plot(-10,-10,110,110,[90,50,10],[90,40,30],[90,50,10],[50,26,20],[90,50,10],[22,13,10])
  dclsbfr : Outport  OutDataType=sfix(16)  OutScaling=2^0  InitialOutput=0
  wires:
  mach/1 -> dcldsbfr/2(Z)
  altitude/1 -> dcldsbfr/1(Y)
  dcldsbfr/1(Interp Value) -> dclsbfr/1

== system gtm_aeromodel/get aero forces and moments/AERODYNAMICS/Aero Incidence Angles/DOWNWASH/eps_spoiler_/epsodsl ==
  Y : Inport  OutDataType=sfix(16)  OutScaling=2^0
  Z : Inport  Port=2  OutDataType=sfix(16)  OutScaling=2^0
  Mux : Mux  Inputs=2
  S-Function : S-Function  FunctionName=table2v5  Parameters=y,z,tab  EnableBusSupport=off
  Interp Value : Outport  OutDataType=sfix(16)  OutScaling=2^0
  wires:
  Z/1 -> Mux/2
  Y/1 -> Mux/1
  S-Function/1 -> Interp Value/1
  Mux/1 -> S-Function/1

== system gtm_aeromodel/get aero forces and moments/AERODYNAMICS/Aero Incidence Angles/DOWNWASH/eps_spoiler_/epsodsl_ ==
  Y : Inport  OutDataType=sfix(16)  OutScaling=2^0
  Z : Inport  Port=2  OutDataType=sfix(16)  OutScaling=2^0
  Mux : Mux  Inputs=2
  S-Function : S-Function  FunctionName=table2v5  Parameters=y,z,tab  EnableBusSupport=off
  Interp Value : Outport  OutDataType=sfix(16)  OutScaling=2^0
  wires:
  Mux/1 -> S-Function/1
  S-Function/1 -> Interp Value/1
  Y/1 -> Mux/1
  Z/1 -> Mux/2

== system gtm_aeromodel/get aero forces and moments/AERODYNAMICS/Aero Incidence Angles/DOWNWASH/eps_spoiler_/epsodsl_1 ==
  Y : Inport  OutDataType=sfix(16)  OutScaling=2^0
  Z : Inport  Port=2  OutDataType=sfix(16)  OutScaling=2^0
  Mux : Mux  Inputs=2
  S-Function : S-Function  FunctionName=table2v5  Parameters=y,z,tab  EnableBusSupport=off
  Interp Value : Outport  OutDataType=sfix(16)  OutScaling=2^0
  wires:
  Z/1 -> Mux/2
  Y/1 -> Mux/1
  S-Function/1 -> Interp Value/1
  Mux/1 -> S-Function/1

== system gtm_aeromodel/get aero forces and moments/AERODYNAMICS/Aero Incidence Angles/DOWNWASH/eps_spoiler_/epsodsl_2 ==
  Y : Inport  OutDataType=sfix(16)  OutScaling=2^0
  Z : Inport  Port=2  OutDataType=sfix(16)  OutScaling=2^0
  Mux : Mux  Inputs=2
  S-Function : S-Function  FunctionName=table2v5  Parameters=y,z,tab  EnableBusSupport=off
  Interp Value : Outport  OutDataType=sfix(16)  OutScaling=2^0
  wires:
  Z/1 -> Mux/2
  Y/1 -> Mux/1
  S-Function/1 -> Interp Value/1
  Mux/1 -> S-Function/1

== system gtm_aeromodel/get aero forces and moments/AERODYNAMICS/Aero Incidence Angles/DOWNWASH/epswb_plus_alphadot/CMAT ==
  Z : Inport  OutDataType=sfix(16)  OutScaling=2^0
  S-Function : S-Function  FunctionName=table1v5  Parameters=z,tab  EnableBusSupport=off
  Interp Value : Outport  OutDataType=sfix(16)  OutScaling=2^0
  wires:
  S-Function/1 -> Interp Value/1
  Z/1 -> S-Function/1

== system gtm_aeromodel/get aero forces and moments/AERODYNAMICS/Aero Incidence Angles/DOWNWASH/epswb_plus_alphadot/clat ==
  Z : Inport  OutDataType=sfix(16)  OutScaling=2^0
  S-Function : S-Function  FunctionName=table1v5  Parameters=z,tab  EnableBusSupport=off
  Interp Value : Outport  OutDataType=sfix(16)  OutScaling=2^0
  wires:
  S-Function/1 -> Interp Value/1
  Z/1 -> S-Function/1
